simulink model "variant"  (R2021b)
settings: Solver=VariableStepAuto  StartTime=0.0  StopTime=10.0  RelTol=1e-3
settings Model: DataDictionary=my_k.sldd  Creator=fredric  LastModifiedBy=fredric

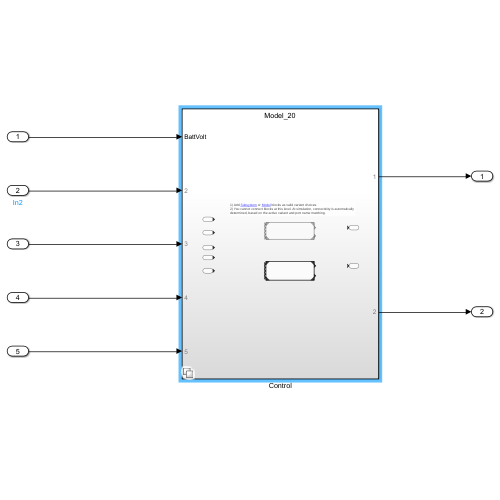
[thumbnail: Simulink's stored preview of the top-level diagram]
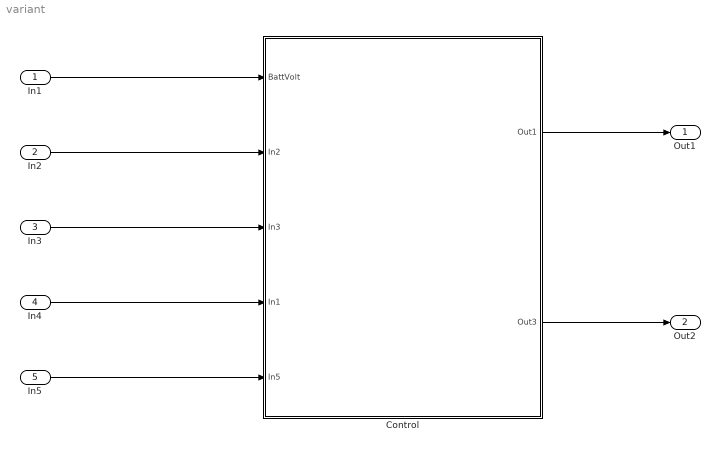
== system variant ==
  In1 : Inport
  In2 : Inport  Port=2
  In3 : Inport  Port=3
  In4 : Inport  Port=4
  In5 : Inport  Port=5
  Control : Subsystem  Variant=on
  Out1 : Outport
  Out2 : Outport  Port=2
  wires:
  In2/1 -> Control/2(In2)
  In4/1 -> Control/4(In1)
  In1/1 -> Control/1(BattVolt)
  In3/1 -> Control/3(In3)
  In5/1 -> Control/5(In5)
  Control/1(Out1) -> Out1/1
  Control/2(Out3) -> Out2/1

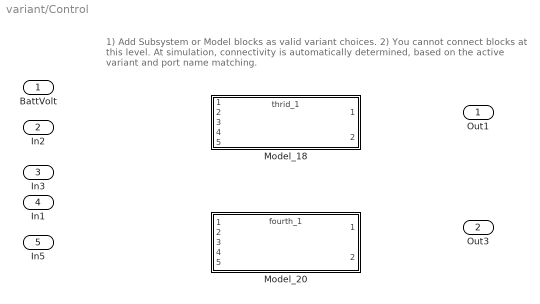
== system variant/Control ==
  note: 1) Add Subsystem or Model blocks as valid variant choices.
      | 2) You cannot connect blocks at this level. At simulation, connectivity is automatically
      | determined, based on the active variant and port name matching.
  BattVolt : Inport
  In2 : Inport  Port=2
  In3 : Inport  Port=3
  In1 : Inport  Port=4
  In5 : Inport  Port=5
  Model_18 : ModelReference  DisableCoverage=on  ModelNameDialog=thrid_1.slx  VariantControl=K == 1  ModelReferenceVersion=1.8
  Model_20 : ModelReference  ModelNameDialog=fourth_1  VariantControl=K == 2  ModelReferenceVersion=1.9
  Out1 : Outport
  Out3 : Outport  Port=2
